simulink model "MTDC_MODEL"  (R2021a)
settings: Solver=ode1  StartTime=0.0  StopTime=3  FixedStep=2e-5  MaxStep=1e-5  RelTol=1e-5  EnableMultiTasking=on
InitFcn:
  | tau_iac=ts_G_iac/4;                                         %Current loop speed
  | wAC=1/tau_iac;                                              %Frequency
  | L1AC=wAC/s;                                                 %Open loop IMC (L) transfer function to obtain a first order after closing the loop
  | Kp_AC=wAC*(Lg_1+La_1/2);                                    %Proportional constant of the controller
  | Ki_AC=wAC*(Rg_1+Ra_1/2);                                    %Integral constant of the controller
  | C_IMC_AC=(Kp_AC*s+Ki_AC)/s;                                 %IMC designed PI controller transfer function
  | TAC=minreal((C_IMC_AC)*G_iac/(1+(C_IMC_AC)*G_iac));         %Closed loop transfer function
  | 
  | tau_Pac=ts_G_P/4;
  | D = TAC*U_ll1;
  | [C_pi,info] = pidtune(D,'PI',1/tau_Pac);
  | Ki_P = C_pi.Ki;
  | 
  | tau_Qac=ts_G_Q/4;
  | [C_piq,info] = pidtune(D,'PI',1/tau_Qac);
  | Ki_Q = C_piq.Ki;
  | 
  | 
  | tau_isum=ts_G_isum/4;                                        %Current loop speed
  | wsum=1/tau_isum;                                             %Frequency
  | L1AC=wsum/s;                                                 %Open loop IMC (L) transfer function to obtain a first order after closing the loop
  | Kp_sum=wsum*(2*La_1);                                        %Proportional constant of the controller
  | Ki_sum=wsum*(2*Ra_1);                                        %Integral constant of the controller
  | C_IMC_sum=(Kp_sum*s+Ki_sum)/s;                               %IMC designed PI controller transfer function
  | 
  | Kp_sum_PR = wc*(2*La_1);
  | Ki_sum_PR = wc*(2*Ra_1);
  | PR = (Kp_sum_PR*s^2 + 2*wc*(Kp_sum_PR+Ki_sum_PR)*s +Kp_sum_PR*w0^2)/(s^2+2*wc*s+w0^2);
  | 
  | 
  | %Energy reference for a converter arm (sum of all the submodule energies)
  | ArmEnergyRef=1/2*Carm*ArmVoltageRef^2;                      %Energy reference for a converter leg
  | LegEnergy=ArmEnergyRef*2;                                   %References for the controllers (DC side)
  | TotalEnergyRef=ArmEnergyRef*6;                              %Reference of the total energy of the converter
  | EnergyDiffabRef=0;                                          %Reference for the energy difference between legs a and b
  | EnergyDiffacRef=0;                                          %Reference for the energy difference between legs b and c
  | 
  | %References for the controllers (AC side)
  | EnergyDiffUpLowRefa=0;                                      %Reference for the energy difference upper and lower arms of phase a
  | EnergyDiffUpLowRefb=0;                                      %Reference for the energy difference upper and lower arms of phase b
  | EnergyDiffUpLowRefc=0;                                      %Reference for the energy difference upper and lower arms of phase c
  |                                                             %Controller design
  | Kpenergy=50;                                                %Proportional gain
  | Kienergy=20;                                                %Integral gain
  | 
  | Kpenergyt=50;                                               %Proportional gain
  | Kienergyt=20;                                               %Integral gain
  | 
  | Q=3;
  | wn=50*2*pi;                                                 %Frequency to eliminate 50 Hz
  | N_50 = tf([1 0 wn^2],[1 2*wn/Q wn^2]);                       %Notch filter 1 design
  | wn=100*2*pi;                                                %Frequency to eliminate 100 Hz
  | N_100 = tf([1 0 wn^2],[1 2*wn/Q wn^2]);                      %Notch filter 2 design
  | Notch=N_50*N_100;                                            %Combination of both notch filters
  | 
  | Ibasedc1= 1000e6/640e3;                 %Nominal current peak DC
  | IsaturationinnerDC1=1.1*Ibasedc1/3;  %Saturation of the DC inner current
  | IsaturationinnerAC1=0.45*Ibasedc1/3; %0.45  %Saturation of the inner current (why edu used 10% - FYI I changed it to 45%)
  | 
  | 
  | ... (+30 lines)
values from neighbouring files (symbols this model uses):
  ArmVoltageRef = 640e3    (= 640000)    [MMC_PARAMETERS.m]
  Cap = 9.5e-3    (= 0.0095)    [MMC_PARAMETERS.m]
  Carm = Cap/N    (= 2.375e-05)    [MMC_PARAMETERS.m]
  f_grid = 50    [MMC_PARAMETERS.m]
  La_1 = 0.15*Zbase_1/2/pi/50    (= 0.0488923985178)    [MMC_PARAMETERS.m]
  Lg_1 = 0.18*Zbase_1/2/pi/50    (= 0.0586708782214)    [MMC_PARAMETERS.m]
  N = 400    [MMC_PARAMETERS.m]
  Ra_1 = 0.01*Zbase_1    (= 1.024)    [MMC_PARAMETERS.m]
  Rg_1 = 0.005*Zbase_1    (= 0.512)    [MMC_PARAMETERS.m]
  S_1 = 1000e6    (= 1000000000)    [MMC_PARAMETERS.m]
  U_ll1 = 320e3    (= 320000)    [MMC_PARAMETERS.m]
  Vdc = 640e3    (= 640000)    [MMC_PARAMETERS.m]
  Vpeak_d1 = U_pnpeak1    [MMC_PARAMETERS.m]
  w0 = 2*pi*50    (= 314.159265359)    [MMC_PARAMETERS.m]
undefined symbols (not defined in the file or in its folder): Kp_Pac, lenght
libraries: spsSeriesRLCBranchLib x80, spsCurrentMeasurementLib x64, spsControlledVoltageSourceLib x36, pid_lib x32, spsVoltageMeasurementLib x32, spsControlledCurrentSourceLib x24, spsParallelRLCBranchLib x20, spsGroundLib x10, powerlib_extras x4, spsDCVoltageSourceLib x4, spspowerguiLib x1
(part 8 of 9)

== system MTDC_MODEL/GRID2+MMC2/Current loop1/Twisting ==
  iq : Inport
  Ref_iq : Inport  Port=2
  Ref_id : Inport  Port=3
  id : Inport  Port=4
  Add : Sum  Inputs=---
  Derivative2 : Derivative
  Gain1 : Gain  Gain=7500
  Gain2 : Gain  Gain=(Rg_1+Ra_1/2)
  Gain4 : Gain  Gain=1000
  Gain5 : Gain  Gain=(Lg_1+La_1/2)
  Gain6 : Gain  Gain=(Lg_1+La_1/2)*2*pi*50
  Scope : Scope  NumInputPorts=2
  Scope1 : Scope  NumInputPorts=2
  Sign : Signum  ZeroCross=off
  Sign1 : Signum  ZeroCross=off
  Sum2 : Sum  Inputs=|++
  Sum5 : Sum  Inputs=|+-
  Out1 : Outport
  Sq : Outport  Port=2
  wires:
  Gain5/1 -> Scope/2, Add/3
  Sign/1 -> Gain4/1
  Gain4/1 -> Sum2/1
  Sum2/1 -> Gain5/1
  Ref_iq/1 -> Gain2/1, Sum5/1
  Gain2/1 -> Add/2
  Gain6/1 -> Add/1
  Add/1 -> Out1/1, Scope/1
  iq/1 -> Sum5/2
  Sum5/1 -> Derivative2/1, Scope1/2, Sq/1, Sign/1  "Sq"
  Ref_id/1 -> Gain6/1
  Sign1/1 -> Gain1/1
  Derivative2/1 -> Sign1/1, Scope1/1
  Gain1/1 -> Sum2/2

== system MTDC_MODEL/GRID2+MMC2/DC References/Sat3 ==
  In1 : Inport
  Demux4 : Demux  Outputs=3
  Mux5 : Mux  Inputs=3
  Saturation1 : Saturate  UpperLimit=IsaturationinnerDC1  LowerLimit=-IsaturationinnerDC1
  Saturation4 : Saturate  UpperLimit=IsaturationinnerDC1  LowerLimit=-IsaturationinnerDC1
  Saturation5 : Saturate  UpperLimit=IsaturationinnerDC1  LowerLimit=-IsaturationinnerDC1
  Out1 : Outport  VectorParamsAs1DForOutWhenUnconnected=off
  wires:
  Saturation5/1 -> Mux5/3
  Saturation4/1 -> Mux5/2
  Saturation1/1 -> Mux5/1
  Demux4/3 -> Saturation5/1
  Demux4/2 -> Saturation4/1
  Demux4/1 -> Saturation1/1
  Mux5/1 -> Out1/1
  In1/1 -> Demux4/1

== system MTDC_MODEL/GRID2+MMC2/Energy Calculation1/AC Power Reference ==
  Ediff_arm_a : Inport
  Ediff_arm_b : Inport  Port=2
  Ediff_arm_c : Inport  Port=3
  Constant1 : Constant  Value=EnergyDiffUpLowRefb
  Constant2 : Constant  Value=EnergyDiffUpLowRefc
  Constant21 : Constant  Value=EnergyDiffUpLowRefa
  PI1 : TransferFcn  Numerator=[Notch.num{1}]  Denominator=[Notch.den{1}]
  PI2 : TransferFcn  Numerator=[Notch.num{1}]  Denominator=[Notch.den{1}]
  PI3 : Subsystem
  PI4 : Subsystem
  PI5 : Subsystem
  PI6 : TransferFcn  Numerator=[Notch.num{1}]  Denominator=[Notch.den{1}]
  Product : Product
  Step : Step  Time=2.1  Before=1  SampleTime=0
  Sum20 : Sum  Inputs=|+-
  Sum21 : Sum  Inputs=|+-
  Sum25 : Sum  Inputs=|+-
  Pdiff_arm_a_Ref : Outport  VectorParamsAs1DForOutWhenUnconnected=off
  Pdiff_arm_b_Ref : Outport  Port=2  VectorParamsAs1DForOutWhenUnconnected=off
  Pdiff_arm_c_Ref : Outport  Port=3  VectorParamsAs1DForOutWhenUnconnected=off
  wires:
  Constant21/1 -> Sum20/1
  Sum25/1 -> PI5/1(e)
  Constant1/1 -> Sum21/1
  Constant2/1 -> Sum25/1
  Sum21/1 -> PI4/1(e)
  Ediff_arm_c/1 -> Sum25/2
  Ediff_arm_a/1 -> Sum20/2
  PI6/1 -> Pdiff_arm_c_Ref/1
  PI5/1(u) -> PI6/1
  PI1/1 -> Pdiff_arm_a_Ref/1
  Sum20/1 -> Product/1
  Ediff_arm_b/1 -> Sum21/2
  PI2/1 -> Pdiff_arm_b_Ref/1
  PI3/1(u) -> PI1/1
  PI4/1(u) -> PI2/1
  Product/1 -> PI3/1(e)
  Step/1 -> Product/2

== system MTDC_MODEL/GRID2+MMC2/Energy Calculation1/DC Energy PIs ==
  EnergyTotal : Inport
  Energydiffab : Inport  Port=2
  Energydiffac : Inport  Port=3
  ACpowerFFd : Inport  Port=4
  DiffabABpowerFFd : Inport  Port=5
  DiffacACpowerFFd : Inport  Port=6
  Constant20 : Constant  Value=TotalEnergyRef
  Constant23 : Constant  Value=EnergyDiffabRef
  Constant29 : Constant  Value=EnergyDiffacRef
  Gain1 : Gain
  Gain43 : Gain
  Gain6 : Gain
  PI1 : TransferFcn  Numerator=[Notch.num{1}]  Denominator=[Notch.den{1}]
  PI10 : TransferFcn  Numerator=[Notch.num{1}]  Denominator=[Notch.den{1}]
  PI2 : TransferFcn  Numerator=[Notch.num{1}]  Denominator=[Notch.den{1}]
  PI3 : TransferFcn  Numerator=[Kpenergyt Kienergyt]  Denominator=[1 0 ]
  PI4 : TransferFcn  Numerator=[Kpenergyt Kienergyt]  Denominator=[1 0 ]
  PI5 : TransferFcn  Numerator=[Kpenergyt Kienergyt]  Denominator=[1 0 ]
  Sum10 : Sum  Inputs=|++
  Sum17 : Sum  Inputs=|++
  Sum20 : Sum  Inputs=|+-
  Sum21 : Sum  Inputs=|+-
  Sum25 : Sum  Inputs=|+-
  Sum27 : Sum  Inputs=|++
  TotalPowerRef : Outport  VectorParamsAs1DForOutWhenUnconnected=off
  DiffabPowerRef : Outport  Port=2  VectorParamsAs1DForOutWhenUnconnected=off
  DiffacPowerRef : Outport  Port=3  VectorParamsAs1DForOutWhenUnconnected=off
  wires:
  Constant20/1 -> Sum20/1
  Sum20/1 -> PI3/1
  Sum25/1 -> PI5/1
  Constant23/1 -> Sum21/1
  Constant29/1 -> Sum25/1
  Sum21/1 -> PI4/1
  PI5/1 -> Gain6/1
  Energydiffab/1 -> Sum21/2
  Energydiffac/1 -> Sum25/2
  EnergyTotal/1 -> Sum20/2
  PI3/1 -> Gain1/1
  PI4/1 -> Gain43/1
  PI2/1 -> DiffabPowerRef/1
  PI10/1 -> DiffacPowerRef/1
  Gain43/1 -> Sum10/1
  Sum17/1 -> PI10/1
  Gain6/1 -> Sum17/1
  Sum10/1 -> PI2/1
  ACpowerFFd/1 -> Sum27/2
  Gain1/1 -> Sum27/1
  PI1/1 -> TotalPowerRef/1
  Sum27/1 -> PI1/1
  DiffacACpowerFFd/1 -> Sum17/2
  DiffabABpowerFFd/1 -> Sum10/2

== system MTDC_MODEL/GRID2+MMC2/Feedforward calculation/First order filter1 ==
  In1 : Inport
  Demux11 : Demux  Outputs=3
  Mux23 : Mux  Inputs=3
  R1 : TransferFcn  Numerator=1  Denominator=[tau_isum 1]
  R2 : TransferFcn  Numerator=1  Denominator=[tau_isum 1]
  R3 : TransferFcn  Numerator=1  Denominator=[tau_isum 1]
  Out1 : Outport  VectorParamsAs1DForOutWhenUnconnected=off
  wires:
  Demux11/2 -> R2/1
  R2/1 -> Mux23/2  "Pub"
  Demux11/1 -> R1/1
  Demux11/3 -> R3/1
  Mux23/1 -> Out1/1
  In1/1 -> Demux11/1
  R3/1 -> Mux23/3  "Puc"
  R1/1 -> Mux23/1  "Pua"

== system MTDC_MODEL/GRID2+MMC2/Isum_AC_Ref_Cal/DIFFERENT_REF_CALC_METHODS  ==
  v_g_pos : Inport
  Constant{1..6} (6 alike) : Constant  Value=0
  Gain1 : Gain  Gain=1/sqrt(2)
  Gain13 : Gain  Gain=1/U_ll1
  Matrix Concatenate4 : Concatenate  NumInputs=3  Mode=Multidimensional array  ConcatenateDimension=2
  Memory : Memory  InitialCondition=Vpeak_d1
  Mux11 : Mux  Inputs=3
  Mux12 : Mux  Inputs=3
  Mux5 : Mux  Inputs=3
  inv mat2 : MATLAB Function  TreatAsAtomicUnit=on
  Initial Approach : Outport  VectorParamsAs1DForOutWhenUnconnected=off
  wires:
  Mux5/1 -> Matrix Concatenate4/3
  Mux11/1 -> Matrix Concatenate4/1
  Constant5/1 -> Mux11/2
  Matrix Concatenate4/1 -> inv mat2/1(u)  "Isum_neg; -Isum_neg;  Isum_pos"
  Constant4/1 -> Mux12/1
  [v_g_pos_rms_pu] -> Mux11/1
  [v_g_pos_rms_pu] -> Mux12/2
  Constant3/1 -> Mux5/2
  [v_g_pos_rms_pu] -> Mux5/3
  inv mat2/1(y) -> Initial Approach/1
  Mux12/1 -> Matrix Concatenate4/2
  Gain1/1 -> [v_g_pos_rms_pu]
  v_g_pos/1 -> Memory/1
  Gain13/1 -> Gain1/1
  Constant1/1 -> Mux11/3
  Constant2/1 -> Mux12/3
  Constant6/1 -> Mux5/1
  Memory/1 -> Gain13/1

== system MTDC_MODEL/GRID2+MMC2/Isum_AC_Ref_Cal/Rotation4 ==
  angle : Inport
  Gain1 : Gain
  Gain2 : Gain  Gain=-1
  Gain9 : Gain  Gain=-1
  Matrix Concatenate1 : Concatenate  Mode=Multidimensional array  ConcatenateDimension=2
  Matrix Concatenate2 : Concatenate  Mode=Multidimensional array  ConcatenateDimension=2
  Mux{1..2,8..9} (4 alike) : Mux  Inputs=2
  Trigonometric Function{1,3..4,6} (4 alike) : Trigonometry  Operator=cos
  Trigonometric Function{2,5,7..8} (4 alike) : Trigonometry
  iR : Outport  VectorParamsAs1DForOutWhenUnconnected=off
  R : Outport  Port=2  VectorParamsAs1DForOutWhenUnconnected=off
  wires:
  Gain2/1 -> Mux2/1
  Matrix Concatenate2/1 -> R/1
  Gain1/1 -> Mux1/2
  Mux2/1 -> Matrix Concatenate2/2
  Mux1/1 -> Matrix Concatenate2/1
  Trigonometric Function8/1 -> Gain2/1
  Trigonometric Function2/1 -> Gain1/1
  Trigonometric Function3/1 -> Mux2/2
  Trigonometric Function1/1 -> Mux1/1
  Matrix Concatenate1/1 -> iR/1
  Gain9/1 -> Mux8/2
  angle/1 -> Trigonometric Function1/1, Trigonometric Function2/1, Trigonometric Function8/1, Trigonometric Function3/1, Trigonometric Function4/1, Trigonometric Function5/1, Trigonometric Function7/1, Trigonometric Function6/1
  Mux9/1 -> Matrix Concatenate1/2
  Mux8/1 -> Matrix Concatenate1/1
  Trigonometric Function7/1 -> Mux9/1
  Trigonometric Function5/1 -> Gain9/1
  Trigonometric Function6/1 -> Mux9/2
  Trigonometric Function4/1 -> Mux8/1

== system MTDC_MODEL/GRID2+MMC2/vsum Calculation/PR Controller1 ==
  e : Inport
  PID Controller2 : pid_lib/PID Controller  Controller=PI  Form=Parallel  TimeDomain=Continuous-time  UseExternalTs=off  SampleTime=1  IntegratorMethod=Forward Euler  FilterMethod=Forward Euler  ControllerParametersSource=internal  P=Kp_sum  I=Ki_sum  D=0  UseFilter=on  N=100  TunerSelectOption=Transfer Function Based (PID Tuner App)  InitialConditionSource=internal  InitialConditionForIntegrator=0  InitialConditionForFilter=0  DifferentiatorICPrevScaledInput=0  ExternalReset=none  TrackingMode=off  Kt=1  LimitOutput=off  SatLimitsSource=internal  UpperSaturationLimit=inf  LowerSaturationLimit=-inf  LinearizeAsGain=on  AntiWindupMode=none  Kb=1  POutMin=[]  POutMax=[]  IOutMin=[]  IOutMax=[]  DOutMin=[]  DOutMax=[]  NOutMin=[]  NOutMax=[]  SumOutMin=[]  SumOutMax=[]  SaturationOutMin=[]  SaturationOutMax=[]  PParamMin=[]  PParamMax=[]  IParamMin=[]  IParamMax=[]  DParamMin=[]  DParamMax=[]  NParamMin=[]  NParamMax=[]  KbParamMin=[]  KbParamMax=[]  KtParamMin=[]  KtParamMax=[]  KbOutMin=[]  KbOutMax=[]  KtOutMin=[]  KtOutMax=[]  IntegratorOutMin=[]  IntegratorOutMax=[]  FilterOutMin=[]  FilterOutMax=[]  SumI1OutMin=[]  SumI1OutMax=[]  SumI2OutMin=[]  SumI2OutMax=[]  SumI3OutMin=[]  SumI3OutMax=[]  SumI4OutMin=[]  SumI4OutMax=[]  SumDOutMin=[]  SumDOutMax=[]  DifferentiatorOutMin=[]  DifferentiatorOutMax=[]  FilterDiffOutCoefMin=[]  FilterDiffOutCoefMax=[]  ReciprocalOutMin=[]  ReciprocalOutMax=[]  SumDenOutMin=[]  SumDenOutMax=[]  SumNumOutMin=[]  SumNumOutMax=[]  DivideOutMin=[]  DivideOutMax=[]  UdiffTsProdOutMin=[]  UdiffTsProdOutMax=[]  NTsProdOutMin=[]  NTsProdOutMax=[]  UintegralTsProdOutMin=[]  UintegralTsProdOutMax=[]  UngainTsProdOutMin=[]  UngainTsProdOutMax=[]  IntegratorContinuousStateAttributes=''  IntegratorStateMustResolveToSignalObject=off  IntegratorRTWStateStorageClass=Auto  FilterContinuousStateAttributes=''  FilterStateMustResolveToSignalObject=off  FilterRTWStateStorageClass=Auto  ParallelPVariant=InternalParameters  IdealPVariant=Disabled  IVariant=InternalParameters  DVariant=Disabled  IntegratorVariant=Continuous  SatVariant=Disabled  AWVariant=Passthrough  PCopyVariant=Disabled  TRVariant=Disabled  FdbkBlocksVariant=Forward  IdealPFdbkVariant=Disabled  SatFdbkVariant=Disabled  DerivativeFilterVariant=Disabled  NVariant=Disabled  NCopyVariant=Disabled_SignalSpec  FilterICVariant=Disabled  IntegratorICVariant=InternalICs  ExternalResetVariant=Disabled  TRSumVariant=Passthrough  SumFdbkVariant=Disabled  SumVariant=Sum_PI  TsampFilterVariant=InternalTs  TsampNgainVariant=Passthrough  TsampIntegralVariant=Passthrough  ExternalSaturationOutDataTypeStr=Inherit: Same as second input
  Sum1 : Sum  Inputs=++|
  Transfer Fcn : TransferFcn  Numerator=PR.num{1}  Denominator=PR.den{1}
  v : Outport
  wires:
  e/1 -> Transfer Fcn/1, PID Controller2/1
  Transfer Fcn/1 -> Sum1/2
  Sum1/1 -> v/1
  PID Controller2/1 -> Sum1/1

== system MTDC_MODEL/GRID2+MMC2/vsum Calculation/PR Controller2 ==
  e : Inport
  PID Controller2 : pid_lib/PID Controller  Controller=PI  Form=Parallel  TimeDomain=Continuous-time  UseExternalTs=off  SampleTime=1  IntegratorMethod=Forward Euler  FilterMethod=Forward Euler  ControllerParametersSource=internal  P=Kp_sum  I=Ki_sum  D=0  UseFilter=on  N=100  TunerSelectOption=Transfer Function Based (PID Tuner App)  InitialConditionSource=internal  InitialConditionForIntegrator=0  InitialConditionForFilter=0  DifferentiatorICPrevScaledInput=0  ExternalReset=none  TrackingMode=off  Kt=1  LimitOutput=off  SatLimitsSource=internal  UpperSaturationLimit=inf  LowerSaturationLimit=-inf  LinearizeAsGain=on  AntiWindupMode=none  Kb=1  POutMin=[]  POutMax=[]  IOutMin=[]  IOutMax=[]  DOutMin=[]  DOutMax=[]  NOutMin=[]  NOutMax=[]  SumOutMin=[]  SumOutMax=[]  SaturationOutMin=[]  SaturationOutMax=[]  PParamMin=[]  PParamMax=[]  IParamMin=[]  IParamMax=[]  DParamMin=[]  DParamMax=[]  NParamMin=[]  NParamMax=[]  KbParamMin=[]  KbParamMax=[]  KtParamMin=[]  KtParamMax=[]  KbOutMin=[]  KbOutMax=[]  KtOutMin=[]  KtOutMax=[]  IntegratorOutMin=[]  IntegratorOutMax=[]  FilterOutMin=[]  FilterOutMax=[]  SumI1OutMin=[]  SumI1OutMax=[]  SumI2OutMin=[]  SumI2OutMax=[]  SumI3OutMin=[]  SumI3OutMax=[]  SumI4OutMin=[]  SumI4OutMax=[]  SumDOutMin=[]  SumDOutMax=[]  DifferentiatorOutMin=[]  DifferentiatorOutMax=[]  FilterDiffOutCoefMin=[]  FilterDiffOutCoefMax=[]  ReciprocalOutMin=[]  ReciprocalOutMax=[]  SumDenOutMin=[]  SumDenOutMax=[]  SumNumOutMin=[]  SumNumOutMax=[]  DivideOutMin=[]  DivideOutMax=[]  UdiffTsProdOutMin=[]  UdiffTsProdOutMax=[]  NTsProdOutMin=[]  NTsProdOutMax=[]  UintegralTsProdOutMin=[]  UintegralTsProdOutMax=[]  UngainTsProdOutMin=[]  UngainTsProdOutMax=[]  IntegratorContinuousStateAttributes=''  IntegratorStateMustResolveToSignalObject=off  IntegratorRTWStateStorageClass=Auto  FilterContinuousStateAttributes=''  FilterStateMustResolveToSignalObject=off  FilterRTWStateStorageClass=Auto  ParallelPVariant=InternalParameters  IdealPVariant=Disabled  IVariant=InternalParameters  DVariant=Disabled  IntegratorVariant=Continuous  SatVariant=Disabled  AWVariant=Passthrough  PCopyVariant=Disabled  TRVariant=Disabled  FdbkBlocksVariant=Forward  IdealPFdbkVariant=Disabled  SatFdbkVariant=Disabled  DerivativeFilterVariant=Disabled  NVariant=Disabled  NCopyVariant=Disabled_SignalSpec  FilterICVariant=Disabled  IntegratorICVariant=InternalICs  ExternalResetVariant=Disabled  TRSumVariant=Passthrough  SumFdbkVariant=Disabled  SumVariant=Sum_PI  TsampFilterVariant=InternalTs  TsampNgainVariant=Passthrough  TsampIntegralVariant=Passthrough  ExternalSaturationOutDataTypeStr=Inherit: Same as second input
  Sum1 : Sum  Inputs=++|
  Transfer Fcn : TransferFcn  Numerator=PR.num{1}  Denominator=PR.den{1}
  v : Outport
  wires:
  PID Controller2/1 -> Sum1/1
  Sum1/1 -> v/1
  Transfer Fcn/1 -> Sum1/2
  e/1 -> PID Controller2/1, Transfer Fcn/1

== system MTDC_MODEL/GRID2+MMC2/vsum Calculation/PR Controller3 ==
  e : Inport
  PID Controller2 : pid_lib/PID Controller  Controller=PI  Form=Parallel  TimeDomain=Continuous-time  UseExternalTs=off  SampleTime=1  IntegratorMethod=Forward Euler  FilterMethod=Forward Euler  ControllerParametersSource=internal  P=Kp_sum  I=Ki_sum  D=0  UseFilter=on  N=100  TunerSelectOption=Transfer Function Based (PID Tuner App)  InitialConditionSource=internal  InitialConditionForIntegrator=0  InitialConditionForFilter=0  DifferentiatorICPrevScaledInput=0  ExternalReset=none  TrackingMode=off  Kt=1  LimitOutput=off  SatLimitsSource=internal  UpperSaturationLimit=inf  LowerSaturationLimit=-inf  LinearizeAsGain=on  AntiWindupMode=none  Kb=1  POutMin=[]  POutMax=[]  IOutMin=[]  IOutMax=[]  DOutMin=[]  DOutMax=[]  NOutMin=[]  NOutMax=[]  SumOutMin=[]  SumOutMax=[]  SaturationOutMin=[]  SaturationOutMax=[]  PParamMin=[]  PParamMax=[]  IParamMin=[]  IParamMax=[]  DParamMin=[]  DParamMax=[]  NParamMin=[]  NParamMax=[]  KbParamMin=[]  KbParamMax=[]  KtParamMin=[]  KtParamMax=[]  KbOutMin=[]  KbOutMax=[]  KtOutMin=[]  KtOutMax=[]  IntegratorOutMin=[]  IntegratorOutMax=[]  FilterOutMin=[]  FilterOutMax=[]  SumI1OutMin=[]  SumI1OutMax=[]  SumI2OutMin=[]  SumI2OutMax=[]  SumI3OutMin=[]  SumI3OutMax=[]  SumI4OutMin=[]  SumI4OutMax=[]  SumDOutMin=[]  SumDOutMax=[]  DifferentiatorOutMin=[]  DifferentiatorOutMax=[]  FilterDiffOutCoefMin=[]  FilterDiffOutCoefMax=[]  ReciprocalOutMin=[]  ReciprocalOutMax=[]  SumDenOutMin=[]  SumDenOutMax=[]  SumNumOutMin=[]  SumNumOutMax=[]  DivideOutMin=[]  DivideOutMax=[]  UdiffTsProdOutMin=[]  UdiffTsProdOutMax=[]  NTsProdOutMin=[]  NTsProdOutMax=[]  UintegralTsProdOutMin=[]  UintegralTsProdOutMax=[]  UngainTsProdOutMin=[]  UngainTsProdOutMax=[]  IntegratorContinuousStateAttributes=''  IntegratorStateMustResolveToSignalObject=off  IntegratorRTWStateStorageClass=Auto  FilterContinuousStateAttributes=''  FilterStateMustResolveToSignalObject=off  FilterRTWStateStorageClass=Auto  ParallelPVariant=InternalParameters  IdealPVariant=Disabled  IVariant=InternalParameters  DVariant=Disabled  IntegratorVariant=Continuous  SatVariant=Disabled  AWVariant=Passthrough  PCopyVariant=Disabled  TRVariant=Disabled  FdbkBlocksVariant=Forward  IdealPFdbkVariant=Disabled  SatFdbkVariant=Disabled  DerivativeFilterVariant=Disabled  NVariant=Disabled  NCopyVariant=Disabled_SignalSpec  FilterICVariant=Disabled  IntegratorICVariant=InternalICs  ExternalResetVariant=Disabled  TRSumVariant=Passthrough  SumFdbkVariant=Disabled  SumVariant=Sum_PI  TsampFilterVariant=InternalTs  TsampNgainVariant=Passthrough  TsampIntegralVariant=Passthrough  ExternalSaturationOutDataTypeStr=Inherit: Same as second input
  Sum1 : Sum  Inputs=++|
  Transfer Fcn : TransferFcn  Numerator=PR.num{1}  Denominator=PR.den{1}
  v : Outport
  wires:
  e/1 -> Transfer Fcn/1, PID Controller2/1
  Transfer Fcn/1 -> Sum1/2
  Sum1/1 -> v/1
  PID Controller2/1 -> Sum1/1

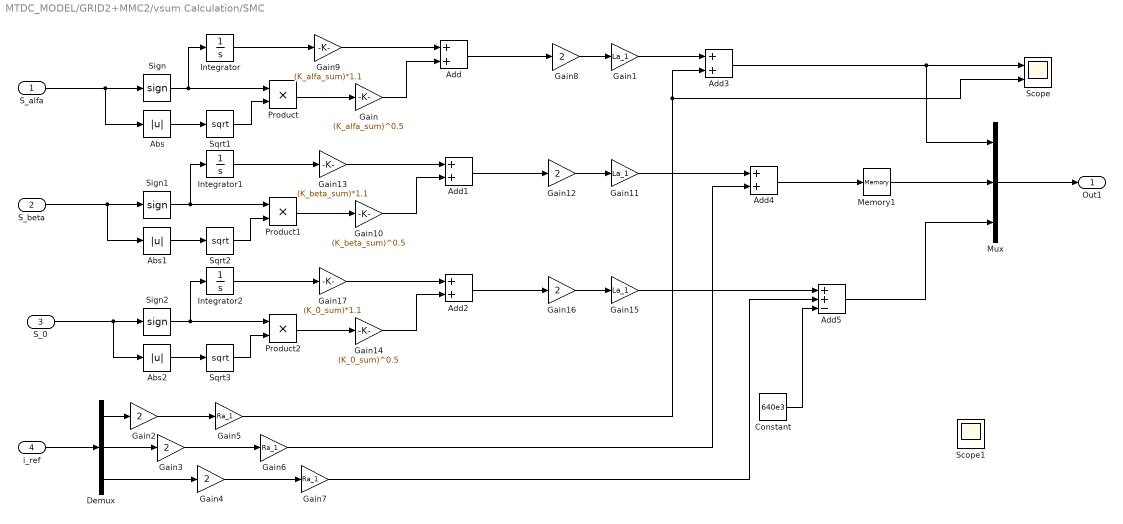
== system MTDC_MODEL/GRID2+MMC2/vsum Calculation/SMC ==
  S_alfa : Inport
  S_beta : Inport  Port=2
  S_0 : Inport  Port=3
  i_ref : Inport  Port=4
  Abs : Abs
  Abs1 : Abs
  Abs2 : Abs
  Add{,1..4} (5 alike) : Sum
  Add5 : Sum  Inputs=++-
  Constant : Constant  Value=640e3
  Demux : Demux  Outputs=3
  Gain : Gain  Gain=(K_alfa_sum)^0.5
  Gain1 : Gain  Gain=La_1
  Gain10 : Gain  Gain=(K_beta_sum)^0.5
  Gain11 : Gain  Gain=La_1
  Gain{2..4,8,12,16} (6 alike) : Gain  Gain=2
  Gain13 : Gain  Gain=(K_beta_sum)*1.1
  Gain14 : Gain  Gain=(K_0_sum)^0.5
  Gain15 : Gain  Gain=La_1
  Gain17 : Gain  Gain=(K_0_sum)*1.1
  Gain5 : Gain  Gain=Ra_1
  Gain6 : Gain  Gain=Ra_1
  Gain7 : Gain  Gain=Ra_1
  Gain9 : Gain  Gain=(K_alfa_sum)*1.1
  Integrator : Integrator
  Integrator1 : Integrator
  Integrator2 : Integrator
  Memory1 : Memory
  Mux : Mux  Inputs=3
  Product : Product
  Product1 : Product
  Product2 : Product
  Scope : Scope  NumInputPorts=2
  Scope1 : Scope
  Sign : Signum
  Sign1 : Signum
  Sign2 : Signum
  Sqrt1 : Sqrt  SaturateOnIntegerOverflow=on
  Sqrt2 : Sqrt  SaturateOnIntegerOverflow=on
  Sqrt3 : Sqrt  SaturateOnIntegerOverflow=on
  Out1 : Outport
  wires:
  i_ref/1 -> Demux/1
  Demux/1 -> Gain2/1
  Demux/2 -> Gain3/1
  Demux/3 -> Gain4/1
  Gain2/1 -> Gain5/1
  Gain3/1 -> Gain6/1
  Gain4/1 -> Gain7/1
  Gain8/1 -> Gain1/1
  S_alfa/1 -> Abs/1, Sign/1
  Sign/1 -> Integrator/1, Product/1
  Product/1 -> Gain/1
  Abs/1 -> Sqrt1/1
  Sqrt1/1 -> Product/2
  Integrator/1 -> Gain9/1
  Gain/1 -> Add/2
  Gain9/1 -> Add/1
  Add/1 -> Gain8/1
  Add1/1 -> Gain12/1
  Gain13/1 -> Add1/1
  Gain10/1 -> Add1/2
  Integrator1/1 -> Gain13/1
  Sqrt2/1 -> Product1/2
  Abs1/1 -> Sqrt2/1
  Product1/1 -> Gain10/1
  Sign1/1 -> Integrator1/1, Product1/1
  S_beta/1 -> Sign1/1, Abs1/1
  Gain12/1 -> Gain11/1
  Gain16/1 -> Gain15/1
  Sign2/1 -> Integrator2/1, Product2/1
  Product2/1 -> Gain14/1
  Abs2/1 -> Sqrt3/1
  Sqrt3/1 -> Product2/2
  Integrator2/1 -> Gain17/1
  Gain14/1 -> Add2/2
  Gain17/1 -> Add2/1
  Add2/1 -> Gain16/1
  Gain6/1 -> Add4/2
  Gain1/1 -> Add3/1
  Gain11/1 -> Add4/1
  Mux/1 -> Out1/1
  Add4/1 -> Memory1/1
  Add5/1 -> Mux/3
  Memory1/1 -> Mux/2
  Gain15/1 -> Add5/1
  Gain7/1 -> Add5/2
  Gain5/1 -> Scope/2, Add3/2
  Add3/1 -> Scope/1, Mux/1
  S_0/1 -> Abs2/1, Sign2/1
  Constant/1 -> Add5/3

== system MTDC_MODEL/GRID3+MMC3/Current loop1/PLCS ==
  iq : Inport
  Ref_iq : Inport  Port=2
  Ref_id : Inport  Port=3
  id : Inport  Port=4
  Abs2 : Abs
  Add : Sum  Inputs=---
  Add1 : Sum
  Constant : Constant  Value=-1/5
  Derivative : Derivative
  Gain1 : Gain  Gain=20000
  Gain14 : Gain  Gain=3900
  Gain2 : Gain  Gain=(Rg_1+Ra_1/2)
  Gain3 : Gain  Gain=(Lg_1+La_1/2)
  Gain6 : Gain  Gain=(Lg_1+La_1/2)*2*pi*50
  Power : Math  Operator=pow  SaturateOnIntegerOverflow=on
  Power1 : Math  Operator=pow  SaturateOnIntegerOverflow=on
  Product : Product
  Scope : Scope  NumInputPorts=2
  Sign1 : Signum
  Sign2 : Signum
  Sqrt3 : Sqrt  SaturateOnIntegerOverflow=on
  Sum5 : Sum  Inputs=|+-
  Out1 : Outport
  Sq : Outport  Port=2
  wires:
  Ref_id/1 -> Gain6/1
  Sum5/1 -> Sign1/1, Scope/2, Sq/1, Derivative/1, Abs2/1  "Sq"
  iq/1 -> Sum5/2
  Add/1 -> Out1/1
  Gain6/1 -> Add/1
  Gain2/1 -> Add/2
  Ref_iq/1 -> Gain2/1, Sum5/1
  Gain3/1 -> Scope/1, Add/3
  Abs2/1 -> Sqrt3/1
  Sign1/1 -> Product/1
  Sqrt3/1 -> Product/2
  Product/1 -> Gain14/1
  Gain14/1 -> Add1/1
  Derivative/1 -> Add1/2
  Add1/1 -> Sign2/1
  Gain1/1 -> Gain3/1
  Sign2/1 -> Gain1/1

== system MTDC_MODEL/GRID3+MMC3/Current loop1/SMC ==
  iq : Inport
  Ref_iq : Inport  Port=2
  Ref_id : Inport  Port=3
  id : Inport  Port=4
  Add : Sum  Inputs=---
  Gain2 : Gain  Gain=(Rg_1+Ra_1/2)
  Gain3 : Gain  Gain=Kq
  Gain4 : Gain  Gain=Qq
  Gain5 : Gain  Gain=(Lg_1+La_1/2)
  Gain6 : Gain  Gain=(Lg_1+La_1/2)*2*pi*50
  Sign : Signum  ZeroCross=off
  Sum2 : Sum  Inputs=|++
  Sum5 : Sum  Inputs=|+-
  Out1 : Outport
  Sq : Outport  Port=2
  wires:
  Sign/1 -> Gain4/1
  Gain3/1 -> Sum2/2
  Gain4/1 -> Sum2/1
  Sum2/1 -> Gain5/1
  Ref_iq/1 -> Gain2/1, Sum5/1
  Gain5/1 -> Add/3
  Gain2/1 -> Add/2
  Gain6/1 -> Add/1
  Add/1 -> Out1/1
  iq/1 -> Sum5/2
  Sum5/1 -> Sq/1, Gain3/1, Sign/1  "Sq"
  Ref_id/1 -> Gain6/1

== system MTDC_MODEL/GRID3+MMC3/Current loop1/SMC1 ==
  id : Inport
  Ref_id : Inport  Port=2
  Ref_iq : Inport  Port=3
  iq : Inport  Port=4
  Add : Sum  Inputs=+--
  Gain2 : Gain  Gain=(Rg_1+Ra_1/2)
  Gain3 : Gain  Gain=Kd
  Gain4 : Gain  Gain=Qd
  Gain5 : Gain  Gain=(Lg_1+La_1/2)
  Gain6 : Gain  Gain=(Lg_1+La_1/2)*2*pi*50
  Sign : Signum  ZeroCross=off
  Sum2 : Sum  Inputs=|++
  Sum5 : Sum  Inputs=|+-
  Out1 : Outport
  Sd : Outport  Port=2
  wires:
  Sum2/1 -> Gain5/1
  Gain4/1 -> Sum2/1
  Gain3/1 -> Sum2/2
  Sign/1 -> Gain4/1
  Ref_id/1 -> Gain2/1, Sum5/1
  Gain6/1 -> Add/1
  Gain2/1 -> Add/2
  Gain5/1 -> Add/3
  id/1 -> Sum5/2
  Sum5/1 -> Sd/1, Gain3/1, Sign/1  "Sd"
  Add/1 -> Out1/1
  Ref_iq/1 -> Gain6/1

== system MTDC_MODEL/GRID3+MMC3/Current loop1/ST-SMC ==
  iq : Inport
  Ref_iq : Inport  Port=2
  Ref_id : Inport  Port=3
  id : Inport  Port=4
  Abs2 : Abs
  Add : Sum  Inputs=---
  Add1 : Sum
  Gain14 : Gain  Gain=4000
  Gain17 : Gain  Gain=4000
  Gain2 : Gain  Gain=(Rg_1+Ra_1/2)
  Gain5 : Gain  Gain=(Lg_1+La_1/2)
  Gain6 : Gain  Gain=(Lg_1+La_1/2)*2*pi*50
  Integrator2 : Integrator
  Product2 : Product
  Scope : Scope  NumInputPorts=2
  Sign2 : Signum
  Sqrt3 : Sqrt  SaturateOnIntegerOverflow=on
  Sum5 : Sum  Inputs=|+-
  Out1 : Outport
  Sq : Outport  Port=2
  wires:
  Gain5/1 -> Scope/2, Add/3
  Ref_iq/1 -> Sum5/1, Gain2/1
  Gain2/1 -> Add/2
  Gain6/1 -> Add/1
  Add/1 -> Scope/1, Out1/1
  iq/1 -> Sum5/2
  Sum5/1 -> Sq/1, Abs2/1, Sign2/1  "Sq"
  Ref_id/1 -> Gain6/1
  Sign2/1 -> Integrator2/1, Product2/1
  Product2/1 -> Gain14/1
  Sqrt3/1 -> Product2/2
  Abs2/1 -> Sqrt3/1
  Integrator2/1 -> Gain17/1
  Add1/1 -> Gain5/1
  Gain17/1 -> Add1/1
  Gain14/1 -> Add1/2

== system MTDC_MODEL/GRID3+MMC3/Current loop1/Twisting ==
  iq : Inport
  Ref_iq : Inport  Port=2
  Ref_id : Inport  Port=3
  id : Inport  Port=4
  Add : Sum  Inputs=---
  Derivative2 : Derivative
  Gain1 : Gain  Gain=7500
  Gain2 : Gain  Gain=(Rg_1+Ra_1/2)
  Gain4 : Gain  Gain=1000
  Gain5 : Gain  Gain=(Lg_1+La_1/2)
  Gain6 : Gain  Gain=(Lg_1+La_1/2)*2*pi*50
  Scope : Scope  NumInputPorts=2
  Scope1 : Scope  NumInputPorts=2
  Sign : Signum  ZeroCross=off
  Sign1 : Signum  ZeroCross=off
  Sum2 : Sum  Inputs=|++
  Sum5 : Sum  Inputs=|+-
  To File1 : ToFile  Filename=sdot2.mat  MatrixName=ans_sdot2  SaveFormat=Timeseries
  To File6 : ToFile  Filename=s2.mat  MatrixName=ans_s2  SaveFormat=Timeseries
  Out1 : Outport
  Sq : Outport  Port=2
  wires:
  Gain5/1 -> Scope/2, Add/3
  Sign/1 -> Gain4/1
  Gain4/1 -> Sum2/1
  Sum2/1 -> Gain5/1
  Ref_iq/1 -> Gain2/1, Sum5/1
  Gain2/1 -> Add/2
  Gain6/1 -> Add/1
  Add/1 -> Out1/1, Scope/1
  iq/1 -> Sum5/2
  Sum5/1 -> Derivative2/1, To File6/1, Scope1/2, Sq/1, Sign/1  "Sq"
  Ref_id/1 -> Gain6/1
  Sign1/1 -> Gain1/1
  Derivative2/1 -> Sign1/1, To File1/1, Scope1/1
  Gain1/1 -> Sum2/2

== system MTDC_MODEL/GRID3+MMC3/DC References/Sat3 ==
  In1 : Inport
  Demux4 : Demux  Outputs=3
  Mux5 : Mux  Inputs=3
  Saturation1 : Saturate  UpperLimit=IsaturationinnerDC1  LowerLimit=-IsaturationinnerDC1
  Saturation4 : Saturate  UpperLimit=IsaturationinnerDC1  LowerLimit=-IsaturationinnerDC1
  Saturation5 : Saturate  UpperLimit=IsaturationinnerDC1  LowerLimit=-IsaturationinnerDC1
  Out1 : Outport  VectorParamsAs1DForOutWhenUnconnected=off
  wires:
  Saturation5/1 -> Mux5/3
  Saturation4/1 -> Mux5/2
  Saturation1/1 -> Mux5/1
  Demux4/3 -> Saturation5/1
  Demux4/2 -> Saturation4/1
  Demux4/1 -> Saturation1/1
  Mux5/1 -> Out1/1
  In1/1 -> Demux4/1

== system MTDC_MODEL/GRID3+MMC3/Energy Calculation1/AC Power Reference ==
  Ediff_arm_a : Inport
  Ediff_arm_b : Inport  Port=2
  Ediff_arm_c : Inport  Port=3
  Constant1 : Constant  Value=EnergyDiffUpLowRefb
  Constant2 : Constant  Value=EnergyDiffUpLowRefc
  Constant21 : Constant  Value=EnergyDiffUpLowRefa
  Mux : Mux  Inputs=3
  PI1 : TransferFcn  Numerator=[Notch.num{1}]  Denominator=[Notch.den{1}]
  PI2 : TransferFcn  Numerator=[Notch.num{1}]  Denominator=[Notch.den{1}]
  PI3 : Subsystem
  PI4 : Subsystem
  PI5 : Subsystem
  PI6 : TransferFcn  Numerator=[Notch.num{1}]  Denominator=[Notch.den{1}]
  Product : Product
  Scope : Scope
  Step : Step  Time=2.1  Before=1  SampleTime=0
  Sum20 : Sum  Inputs=|+-
  Sum21 : Sum  Inputs=|+-
  Sum25 : Sum  Inputs=|+-
  Pdiff_arm_a_Ref : Outport  VectorParamsAs1DForOutWhenUnconnected=off
  Pdiff_arm_b_Ref : Outport  Port=2  VectorParamsAs1DForOutWhenUnconnected=off
  Pdiff_arm_c_Ref : Outport  Port=3  VectorParamsAs1DForOutWhenUnconnected=off
  wires:
  Constant21/1 -> Sum20/1
  Sum25/1 -> PI5/1(e)
  Constant1/1 -> Sum21/1
  Constant2/1 -> Sum25/1
  Sum21/1 -> PI4/1(e)
  Ediff_arm_c/1 -> Mux/3, Sum25/2
  Ediff_arm_a/1 -> Mux/1, Sum20/2
  PI6/1 -> Pdiff_arm_c_Ref/1
  PI5/1(u) -> PI6/1
  PI1/1 -> Pdiff_arm_a_Ref/1
  Sum20/1 -> Product/1
  Ediff_arm_b/1 -> Mux/2, Sum21/2
  PI2/1 -> Pdiff_arm_b_Ref/1
  PI3/1(u) -> PI1/1
  PI4/1(u) -> PI2/1
  Product/1 -> PI3/1(e)
  Step/1 -> Product/2
  Mux/1 -> Scope/1

== system MTDC_MODEL/GRID3+MMC3/Energy Calculation1/DC Energy PIs ==
  EnergyTotal : Inport
  Energydiffab : Inport  Port=2
  Energydiffac : Inport  Port=3
  ACpowerFFd : Inport  Port=4
  DiffabABpowerFFd : Inport  Port=5
  DiffacACpowerFFd : Inport  Port=6
  Constant20 : Constant  Value=TotalEnergyRef
  Constant23 : Constant  Value=EnergyDiffabRef
  Constant29 : Constant  Value=EnergyDiffacRef
  Gain1 : Gain
  Gain43 : Gain
  Gain6 : Gain
  Mux : Mux  Inputs=2
  PI1 : TransferFcn  Numerator=[Notch.num{1}]  Denominator=[Notch.den{1}]
  PI10 : TransferFcn  Numerator=[Notch.num{1}]  Denominator=[Notch.den{1}]
  PI2 : TransferFcn  Numerator=[Notch.num{1}]  Denominator=[Notch.den{1}]
  PI3 : TransferFcn  Numerator=[Kpenergyt Kienergyt]  Denominator=[1 0 ]
  PI4 : TransferFcn  Numerator=[Kpenergyt Kienergyt]  Denominator=[1 0 ]
  PI5 : TransferFcn  Numerator=[Kpenergyt Kienergyt]  Denominator=[1 0 ]
  Scope : Scope
  Sum10 : Sum  Inputs=|++
  Sum17 : Sum  Inputs=|++
  Sum20 : Sum  Inputs=|+-
  Sum21 : Sum  Inputs=|+-
  Sum25 : Sum  Inputs=|+-
  Sum27 : Sum  Inputs=|++
  TotalPowerRef : Outport  VectorParamsAs1DForOutWhenUnconnected=off
  DiffabPowerRef : Outport  Port=2  VectorParamsAs1DForOutWhenUnconnected=off
  DiffacPowerRef : Outport  Port=3  VectorParamsAs1DForOutWhenUnconnected=off
  wires:
  Constant20/1 -> Sum20/1
  Sum20/1 -> PI3/1
  Sum25/1 -> PI5/1
  Constant23/1 -> Sum21/1
  Constant29/1 -> Sum25/1
  Sum21/1 -> PI4/1
  PI5/1 -> Gain6/1
  Energydiffab/1 -> Mux/1, Sum21/2
  Energydiffac/1 -> Mux/2, Sum25/2
  EnergyTotal/1 -> Sum20/2
  PI3/1 -> Gain1/1
  PI4/1 -> Gain43/1
  PI2/1 -> DiffabPowerRef/1
  PI10/1 -> DiffacPowerRef/1
  Gain43/1 -> Sum10/1
  Sum17/1 -> PI10/1
  Gain6/1 -> Sum17/1
  Sum10/1 -> PI2/1
  ACpowerFFd/1 -> Sum27/2
  Gain1/1 -> Sum27/1
  PI1/1 -> TotalPowerRef/1
  Sum27/1 -> PI1/1
  DiffacACpowerFFd/1 -> Sum17/2
  DiffabABpowerFFd/1 -> Sum10/2
  Mux/1 -> Scope/1

== system MTDC_MODEL/GRID3+MMC3/Feedforward calculation/First order filter1 ==
  In1 : Inport
  Demux11 : Demux  Outputs=3
  Mux23 : Mux  Inputs=3
  R1 : TransferFcn  Numerator=1  Denominator=[tau_isum 1]
  R2 : TransferFcn  Numerator=1  Denominator=[tau_isum 1]
  R3 : TransferFcn  Numerator=1  Denominator=[tau_isum 1]
  Out1 : Outport  VectorParamsAs1DForOutWhenUnconnected=off
  wires:
  Demux11/2 -> R2/1
  R2/1 -> Mux23/2  "Pub"
  Demux11/1 -> R1/1
  Demux11/3 -> R3/1
  Mux23/1 -> Out1/1
  In1/1 -> Demux11/1
  R3/1 -> Mux23/3  "Puc"
  R1/1 -> Mux23/1  "Pua"

== system MTDC_MODEL/GRID3+MMC3/Isum_AC_Ref_Cal/DIFFERENT_REF_CALC_METHODS  ==
  v_g_pos : Inport
  Constant{1..6} (6 alike) : Constant  Value=0
  Gain1 : Gain  Gain=1/sqrt(2)
  Gain13 : Gain  Gain=1/U_ll1
  Matrix Concatenate4 : Concatenate  NumInputs=3  Mode=Multidimensional array  ConcatenateDimension=2
  Memory : Memory  InitialCondition=Vpeak_d1
  Mux11 : Mux  Inputs=3
  Mux12 : Mux  Inputs=3
  Mux5 : Mux  Inputs=3
  inv mat2 : MATLAB Function  TreatAsAtomicUnit=on
  Initial Approach : Outport  VectorParamsAs1DForOutWhenUnconnected=off
  wires:
  Mux5/1 -> Matrix Concatenate4/3
  Mux11/1 -> Matrix Concatenate4/1
  Constant5/1 -> Mux11/2
  Matrix Concatenate4/1 -> inv mat2/1(u)  "Isum_neg; -Isum_neg;  Isum_pos"
  Constant4/1 -> Mux12/1
  [v_g_pos_rms_pu] -> Mux11/1
  [v_g_pos_rms_pu] -> Mux12/2
  Constant3/1 -> Mux5/2
  [v_g_pos_rms_pu] -> Mux5/3
  inv mat2/1(y) -> Initial Approach/1
  Mux12/1 -> Matrix Concatenate4/2
  Gain1/1 -> [v_g_pos_rms_pu]
  v_g_pos/1 -> Memory/1
  Gain13/1 -> Gain1/1
  Constant1/1 -> Mux11/3
  Constant2/1 -> Mux12/3
  Constant6/1 -> Mux5/1
  Memory/1 -> Gain13/1

== system MTDC_MODEL/GRID3+MMC3/Isum_AC_Ref_Cal/Rotation4 ==
  angle : Inport
  Gain1 : Gain
  Gain2 : Gain  Gain=-1
  Gain9 : Gain  Gain=-1
  Matrix Concatenate1 : Concatenate  Mode=Multidimensional array  ConcatenateDimension=2
  Matrix Concatenate2 : Concatenate  Mode=Multidimensional array  ConcatenateDimension=2
  Mux{1..2,8..9} (4 alike) : Mux  Inputs=2
  Trigonometric Function{1,3..4,6} (4 alike) : Trigonometry  Operator=cos
  Trigonometric Function{2,5,7..8} (4 alike) : Trigonometry
  iR : Outport  VectorParamsAs1DForOutWhenUnconnected=off
  R : Outport  Port=2  VectorParamsAs1DForOutWhenUnconnected=off
  wires:
  Gain2/1 -> Mux2/1
  Matrix Concatenate2/1 -> R/1
  Gain1/1 -> Mux1/2
  Mux2/1 -> Matrix Concatenate2/2
  Mux1/1 -> Matrix Concatenate2/1
  Trigonometric Function8/1 -> Gain2/1
  Trigonometric Function2/1 -> Gain1/1
  Trigonometric Function3/1 -> Mux2/2
  Trigonometric Function1/1 -> Mux1/1
  Matrix Concatenate1/1 -> iR/1
  Gain9/1 -> Mux8/2
  angle/1 -> Trigonometric Function1/1, Trigonometric Function2/1, Trigonometric Function8/1, Trigonometric Function3/1, Trigonometric Function4/1, Trigonometric Function5/1, Trigonometric Function7/1, Trigonometric Function6/1
  Mux9/1 -> Matrix Concatenate1/2
  Mux8/1 -> Matrix Concatenate1/1
  Trigonometric Function7/1 -> Mux9/1
  Trigonometric Function5/1 -> Gain9/1
  Trigonometric Function6/1 -> Mux9/2
  Trigonometric Function4/1 -> Mux8/1

== system MTDC_MODEL/GRID3+MMC3/vsum Calculation/PR Controller1 ==
  e : Inport
  PID Controller2 : pid_lib/PID Controller  Controller=PI  Form=Parallel  TimeDomain=Continuous-time  UseExternalTs=off  SampleTime=1  IntegratorMethod=Forward Euler  FilterMethod=Forward Euler  ControllerParametersSource=internal  P=Kp_sum  I=Ki_sum  D=0  UseFilter=on  N=100  TunerSelectOption=Transfer Function Based (PID Tuner App)  InitialConditionSource=internal  InitialConditionForIntegrator=0  InitialConditionForFilter=0  DifferentiatorICPrevScaledInput=0  ExternalReset=none  TrackingMode=off  Kt=1  LimitOutput=off  SatLimitsSource=internal  UpperSaturationLimit=inf  LowerSaturationLimit=-inf  LinearizeAsGain=on  AntiWindupMode=none  Kb=1  POutMin=[]  POutMax=[]  IOutMin=[]  IOutMax=[]  DOutMin=[]  DOutMax=[]  NOutMin=[]  NOutMax=[]  SumOutMin=[]  SumOutMax=[]  SaturationOutMin=[]  SaturationOutMax=[]  PParamMin=[]  PParamMax=[]  IParamMin=[]  IParamMax=[]  DParamMin=[]  DParamMax=[]  NParamMin=[]  NParamMax=[]  KbParamMin=[]  KbParamMax=[]  KtParamMin=[]  KtParamMax=[]  KbOutMin=[]  KbOutMax=[]  KtOutMin=[]  KtOutMax=[]  IntegratorOutMin=[]  IntegratorOutMax=[]  FilterOutMin=[]  FilterOutMax=[]  SumI1OutMin=[]  SumI1OutMax=[]  SumI2OutMin=[]  SumI2OutMax=[]  SumI3OutMin=[]  SumI3OutMax=[]  SumI4OutMin=[]  SumI4OutMax=[]  SumDOutMin=[]  SumDOutMax=[]  DifferentiatorOutMin=[]  DifferentiatorOutMax=[]  FilterDiffOutCoefMin=[]  FilterDiffOutCoefMax=[]  ReciprocalOutMin=[]  ReciprocalOutMax=[]  SumDenOutMin=[]  SumDenOutMax=[]  SumNumOutMin=[]  SumNumOutMax=[]  DivideOutMin=[]  DivideOutMax=[]  UdiffTsProdOutMin=[]  UdiffTsProdOutMax=[]  NTsProdOutMin=[]  NTsProdOutMax=[]  UintegralTsProdOutMin=[]  UintegralTsProdOutMax=[]  UngainTsProdOutMin=[]  UngainTsProdOutMax=[]  IntegratorContinuousStateAttributes=''  IntegratorStateMustResolveToSignalObject=off  IntegratorRTWStateStorageClass=Auto  FilterContinuousStateAttributes=''  FilterStateMustResolveToSignalObject=off  FilterRTWStateStorageClass=Auto  ParallelPVariant=InternalParameters  IdealPVariant=Disabled  IVariant=InternalParameters  DVariant=Disabled  IntegratorVariant=Continuous  SatVariant=Disabled  AWVariant=Passthrough  PCopyVariant=Disabled  TRVariant=Disabled  FdbkBlocksVariant=Forward  IdealPFdbkVariant=Disabled  SatFdbkVariant=Disabled  DerivativeFilterVariant=Disabled  NVariant=Disabled  NCopyVariant=Disabled_SignalSpec  FilterICVariant=Disabled  IntegratorICVariant=InternalICs  ExternalResetVariant=Disabled  TRSumVariant=Passthrough  SumFdbkVariant=Disabled  SumVariant=Sum_PI  TsampFilterVariant=InternalTs  TsampNgainVariant=Passthrough  TsampIntegralVariant=Passthrough  ExternalSaturationOutDataTypeStr=Inherit: Same as second input
  Sum1 : Sum  Inputs=++|
  Transfer Fcn : TransferFcn  Numerator=PR.num{1}  Denominator=PR.den{1}
  v : Outport
  wires:
  e/1 -> Transfer Fcn/1, PID Controller2/1
  Transfer Fcn/1 -> Sum1/2
  Sum1/1 -> v/1
  PID Controller2/1 -> Sum1/1

== system MTDC_MODEL/GRID3+MMC3/vsum Calculation/PR Controller2 ==
  e : Inport
  PID Controller2 : pid_lib/PID Controller  Controller=PI  Form=Parallel  TimeDomain=Continuous-time  UseExternalTs=off  SampleTime=1  IntegratorMethod=Forward Euler  FilterMethod=Forward Euler  ControllerParametersSource=internal  P=Kp_sum  I=Ki_sum  D=0  UseFilter=on  N=100  TunerSelectOption=Transfer Function Based (PID Tuner App)  InitialConditionSource=internal  InitialConditionForIntegrator=0  InitialConditionForFilter=0  DifferentiatorICPrevScaledInput=0  ExternalReset=none  TrackingMode=off  Kt=1  LimitOutput=off  SatLimitsSource=internal  UpperSaturationLimit=inf  LowerSaturationLimit=-inf  LinearizeAsGain=on  AntiWindupMode=none  Kb=1  POutMin=[]  POutMax=[]  IOutMin=[]  IOutMax=[]  DOutMin=[]  DOutMax=[]  NOutMin=[]  NOutMax=[]  SumOutMin=[]  SumOutMax=[]  SaturationOutMin=[]  SaturationOutMax=[]  PParamMin=[]  PParamMax=[]  IParamMin=[]  IParamMax=[]  DParamMin=[]  DParamMax=[]  NParamMin=[]  NParamMax=[]  KbParamMin=[]  KbParamMax=[]  KtParamMin=[]  KtParamMax=[]  KbOutMin=[]  KbOutMax=[]  KtOutMin=[]  KtOutMax=[]  IntegratorOutMin=[]  IntegratorOutMax=[]  FilterOutMin=[]  FilterOutMax=[]  SumI1OutMin=[]  SumI1OutMax=[]  SumI2OutMin=[]  SumI2OutMax=[]  SumI3OutMin=[]  SumI3OutMax=[]  SumI4OutMin=[]  SumI4OutMax=[]  SumDOutMin=[]  SumDOutMax=[]  DifferentiatorOutMin=[]  DifferentiatorOutMax=[]  FilterDiffOutCoefMin=[]  FilterDiffOutCoefMax=[]  ReciprocalOutMin=[]  ReciprocalOutMax=[]  SumDenOutMin=[]  SumDenOutMax=[]  SumNumOutMin=[]  SumNumOutMax=[]  DivideOutMin=[]  DivideOutMax=[]  UdiffTsProdOutMin=[]  UdiffTsProdOutMax=[]  NTsProdOutMin=[]  NTsProdOutMax=[]  UintegralTsProdOutMin=[]  UintegralTsProdOutMax=[]  UngainTsProdOutMin=[]  UngainTsProdOutMax=[]  IntegratorContinuousStateAttributes=''  IntegratorStateMustResolveToSignalObject=off  IntegratorRTWStateStorageClass=Auto  FilterContinuousStateAttributes=''  FilterStateMustResolveToSignalObject=off  FilterRTWStateStorageClass=Auto  ParallelPVariant=InternalParameters  IdealPVariant=Disabled  IVariant=InternalParameters  DVariant=Disabled  IntegratorVariant=Continuous  SatVariant=Disabled  AWVariant=Passthrough  PCopyVariant=Disabled  TRVariant=Disabled  FdbkBlocksVariant=Forward  IdealPFdbkVariant=Disabled  SatFdbkVariant=Disabled  DerivativeFilterVariant=Disabled  NVariant=Disabled  NCopyVariant=Disabled_SignalSpec  FilterICVariant=Disabled  IntegratorICVariant=InternalICs  ExternalResetVariant=Disabled  TRSumVariant=Passthrough  SumFdbkVariant=Disabled  SumVariant=Sum_PI  TsampFilterVariant=InternalTs  TsampNgainVariant=Passthrough  TsampIntegralVariant=Passthrough  ExternalSaturationOutDataTypeStr=Inherit: Same as second input
  Sum1 : Sum  Inputs=++|
  Transfer Fcn : TransferFcn  Numerator=PR.num{1}  Denominator=PR.den{1}
  v : Outport
  wires:
  PID Controller2/1 -> Sum1/1
  Sum1/1 -> v/1
  Transfer Fcn/1 -> Sum1/2
  e/1 -> PID Controller2/1, Transfer Fcn/1

== system MTDC_MODEL/GRID3+MMC3/vsum Calculation/PR Controller3 ==
  e : Inport
  PID Controller2 : pid_lib/PID Controller  Controller=PI  Form=Parallel  TimeDomain=Continuous-time  UseExternalTs=off  SampleTime=1  IntegratorMethod=Forward Euler  FilterMethod=Forward Euler  ControllerParametersSource=internal  P=Kp_sum  I=Ki_sum  D=0  UseFilter=on  N=100  TunerSelectOption=Transfer Function Based (PID Tuner App)  InitialConditionSource=internal  InitialConditionForIntegrator=0  InitialConditionForFilter=0  DifferentiatorICPrevScaledInput=0  ExternalReset=none  TrackingMode=off  Kt=1  LimitOutput=off  SatLimitsSource=internal  UpperSaturationLimit=inf  LowerSaturationLimit=-inf  LinearizeAsGain=on  AntiWindupMode=none  Kb=1  POutMin=[]  POutMax=[]  IOutMin=[]  IOutMax=[]  DOutMin=[]  DOutMax=[]  NOutMin=[]  NOutMax=[]  SumOutMin=[]  SumOutMax=[]  SaturationOutMin=[]  SaturationOutMax=[]  PParamMin=[]  PParamMax=[]  IParamMin=[]  IParamMax=[]  DParamMin=[]  DParamMax=[]  NParamMin=[]  NParamMax=[]  KbParamMin=[]  KbParamMax=[]  KtParamMin=[]  KtParamMax=[]  KbOutMin=[]  KbOutMax=[]  KtOutMin=[]  KtOutMax=[]  IntegratorOutMin=[]  IntegratorOutMax=[]  FilterOutMin=[]  FilterOutMax=[]  SumI1OutMin=[]  SumI1OutMax=[]  SumI2OutMin=[]  SumI2OutMax=[]  SumI3OutMin=[]  SumI3OutMax=[]  SumI4OutMin=[]  SumI4OutMax=[]  SumDOutMin=[]  SumDOutMax=[]  DifferentiatorOutMin=[]  DifferentiatorOutMax=[]  FilterDiffOutCoefMin=[]  FilterDiffOutCoefMax=[]  ReciprocalOutMin=[]  ReciprocalOutMax=[]  SumDenOutMin=[]  SumDenOutMax=[]  SumNumOutMin=[]  SumNumOutMax=[]  DivideOutMin=[]  DivideOutMax=[]  UdiffTsProdOutMin=[]  UdiffTsProdOutMax=[]  NTsProdOutMin=[]  NTsProdOutMax=[]  UintegralTsProdOutMin=[]  UintegralTsProdOutMax=[]  UngainTsProdOutMin=[]  UngainTsProdOutMax=[]  IntegratorContinuousStateAttributes=''  IntegratorStateMustResolveToSignalObject=off  IntegratorRTWStateStorageClass=Auto  FilterContinuousStateAttributes=''  FilterStateMustResolveToSignalObject=off  FilterRTWStateStorageClass=Auto  ParallelPVariant=InternalParameters  IdealPVariant=Disabled  IVariant=InternalParameters  DVariant=Disabled  IntegratorVariant=Continuous  SatVariant=Disabled  AWVariant=Passthrough  PCopyVariant=Disabled  TRVariant=Disabled  FdbkBlocksVariant=Forward  IdealPFdbkVariant=Disabled  SatFdbkVariant=Disabled  DerivativeFilterVariant=Disabled  NVariant=Disabled  NCopyVariant=Disabled_SignalSpec  FilterICVariant=Disabled  IntegratorICVariant=InternalICs  ExternalResetVariant=Disabled  TRSumVariant=Passthrough  SumFdbkVariant=Disabled  SumVariant=Sum_PI  TsampFilterVariant=InternalTs  TsampNgainVariant=Passthrough  TsampIntegralVariant=Passthrough  ExternalSaturationOutDataTypeStr=Inherit: Same as second input
  Sum1 : Sum  Inputs=++|
  Transfer Fcn : TransferFcn  Numerator=PR.num{1}  Denominator=PR.den{1}
  v : Outport
  wires:
  e/1 -> Transfer Fcn/1, PID Controller2/1
  Transfer Fcn/1 -> Sum1/2
  Sum1/1 -> v/1
  PID Controller2/1 -> Sum1/1

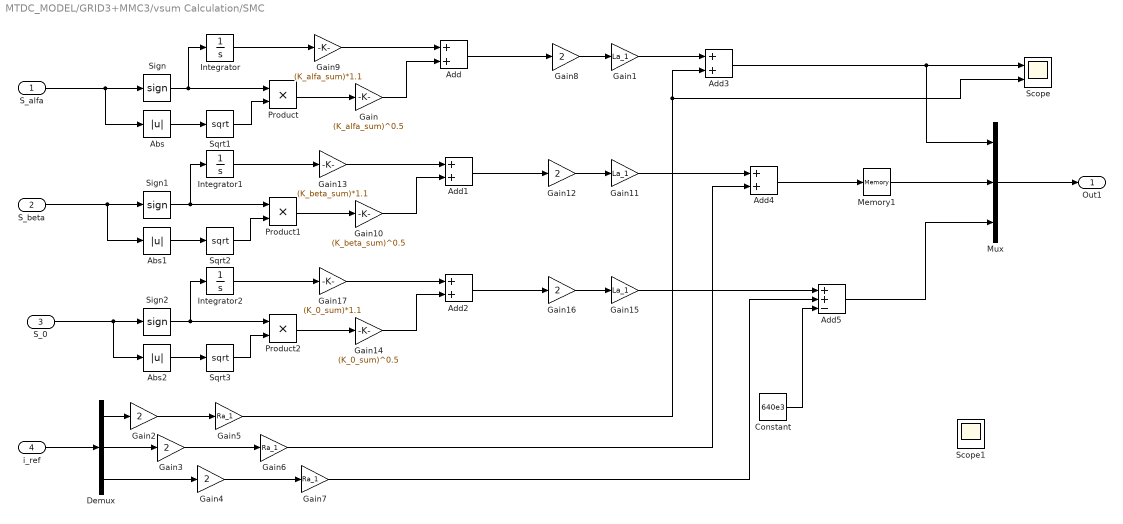
== system MTDC_MODEL/GRID3+MMC3/vsum Calculation/SMC ==
  S_alfa : Inport
  S_beta : Inport  Port=2
  S_0 : Inport  Port=3
  i_ref : Inport  Port=4
  Abs : Abs
  Abs1 : Abs
  Abs2 : Abs
  Add{,1..4} (5 alike) : Sum
  Add5 : Sum  Inputs=++-
  Constant : Constant  Value=640e3
  Demux : Demux  Outputs=3
  Gain : Gain  Gain=(K_alfa_sum)^0.5
  Gain1 : Gain  Gain=La_1
  Gain10 : Gain  Gain=(K_beta_sum)^0.5
  Gain11 : Gain  Gain=La_1
  Gain{2..4,8,12,16} (6 alike) : Gain  Gain=2
  Gain13 : Gain  Gain=(K_beta_sum)*1.1
  Gain14 : Gain  Gain=(K_0_sum)^0.5
  Gain15 : Gain  Gain=La_1
  Gain17 : Gain  Gain=(K_0_sum)*1.1
  Gain5 : Gain  Gain=Ra_1
  Gain6 : Gain  Gain=Ra_1
  Gain7 : Gain  Gain=Ra_1
  Gain9 : Gain  Gain=(K_alfa_sum)*1.1
  Integrator : Integrator
  Integrator1 : Integrator
  Integrator2 : Integrator
  Memory1 : Memory
  Mux : Mux  Inputs=3
  Product : Product
  Product1 : Product
  Product2 : Product
  Scope : Scope  NumInputPorts=2
  Scope1 : Scope
  Sign : Signum
  Sign1 : Signum
  Sign2 : Signum
  Sqrt1 : Sqrt  SaturateOnIntegerOverflow=on
  Sqrt2 : Sqrt  SaturateOnIntegerOverflow=on
  Sqrt3 : Sqrt  SaturateOnIntegerOverflow=on
  Out1 : Outport
  wires:
  i_ref/1 -> Demux/1
  Demux/1 -> Gain2/1
  Demux/2 -> Gain3/1
  Demux/3 -> Gain4/1
  Gain2/1 -> Gain5/1
  Gain3/1 -> Gain6/1
  Gain4/1 -> Gain7/1
  Gain8/1 -> Gain1/1
  S_alfa/1 -> Abs/1, Sign/1
  Sign/1 -> Integrator/1, Product/1
  Product/1 -> Gain/1
  Abs/1 -> Sqrt1/1
  Sqrt1/1 -> Product/2
  Integrator/1 -> Gain9/1
  Gain/1 -> Add/2
  Gain9/1 -> Add/1
  Add/1 -> Gain8/1
  Add1/1 -> Gain12/1
  Gain13/1 -> Add1/1
  Gain10/1 -> Add1/2
  Integrator1/1 -> Gain13/1
  Sqrt2/1 -> Product1/2
  Abs1/1 -> Sqrt2/1
  Product1/1 -> Gain10/1
  Sign1/1 -> Integrator1/1, Product1/1
  S_beta/1 -> Sign1/1, Abs1/1
  Gain12/1 -> Gain11/1
  Gain16/1 -> Gain15/1
  Sign2/1 -> Integrator2/1, Product2/1
  Product2/1 -> Gain14/1
  Abs2/1 -> Sqrt3/1
  Sqrt3/1 -> Product2/2
  Integrator2/1 -> Gain17/1
  Gain14/1 -> Add2/2
  Gain17/1 -> Add2/1
  Add2/1 -> Gain16/1
  Gain6/1 -> Add4/2
  Gain1/1 -> Add3/1
  Gain11/1 -> Add4/1
  Mux/1 -> Out1/1
  Add4/1 -> Memory1/1
  Add5/1 -> Mux/3
  Memory1/1 -> Mux/2
  Gain15/1 -> Add5/1
  Gain7/1 -> Add5/2
  Gain5/1 -> Scope/2, Add3/2
  Add3/1 -> Scope/1, Mux/1
  S_0/1 -> Abs2/1, Sign2/1
  Constant/1 -> Add5/3

== system MTDC_MODEL/GRID4+MMC4/Current loop1/PLCS ==
  iq : Inport
  Ref_iq : Inport  Port=2
  Ref_id : Inport  Port=3
  id : Inport  Port=4
  Abs2 : Abs
  Add : Sum  Inputs=---
  Add1 : Sum
  Constant : Constant  Value=-1/5
  Derivative : Derivative
  Gain1 : Gain  Gain=20000
  Gain14 : Gain  Gain=3900
  Gain2 : Gain  Gain=(Rg_1+Ra_1/2)
  Gain3 : Gain  Gain=(Lg_1+La_1/2)
  Gain6 : Gain  Gain=(Lg_1+La_1/2)*2*pi*50
  Power : Math  Operator=pow  SaturateOnIntegerOverflow=on
  Power1 : Math  Operator=pow  SaturateOnIntegerOverflow=on
  Product : Product
  Scope : Scope  NumInputPorts=2
  Sign1 : Signum
  Sign2 : Signum
  Sqrt3 : Sqrt  SaturateOnIntegerOverflow=on
  Sum5 : Sum  Inputs=|+-
  Out1 : Outport
  Sq : Outport  Port=2
  wires:
  Ref_id/1 -> Gain6/1
  Sum5/1 -> Sign1/1, Scope/2, Sq/1, Derivative/1, Abs2/1  "Sq"
  iq/1 -> Sum5/2
  Add/1 -> Out1/1
  Gain6/1 -> Add/1
  Gain2/1 -> Add/2
  Ref_iq/1 -> Gain2/1, Sum5/1
  Gain3/1 -> Scope/1, Add/3
  Abs2/1 -> Sqrt3/1
  Sign1/1 -> Product/1
  Sqrt3/1 -> Product/2
  Product/1 -> Gain14/1
  Gain14/1 -> Add1/1
  Derivative/1 -> Add1/2
  Add1/1 -> Sign2/1
  Gain1/1 -> Gain3/1
  Sign2/1 -> Gain1/1

== system MTDC_MODEL/GRID4+MMC4/Current loop1/SMC ==
  iq : Inport
  Ref_iq : Inport  Port=2
  Ref_id : Inport  Port=3
  id : Inport  Port=4
  Add : Sum  Inputs=---
  Gain2 : Gain  Gain=(Rg_1+Ra_1/2)
  Gain3 : Gain  Gain=Kq
  Gain4 : Gain  Gain=Qq
  Gain5 : Gain  Gain=(Lg_1+La_1/2)
  Gain6 : Gain  Gain=(Lg_1+La_1/2)*2*pi*50
  Sign : Signum  ZeroCross=off
  Sum2 : Sum  Inputs=|++
  Sum5 : Sum  Inputs=|+-
  Out1 : Outport
  wires:
  Ref_id/1 -> Gain6/1
  Sum5/1 -> Sign/1, Gain3/1  "Sq"
  iq/1 -> Sum5/2
  Add/1 -> Out1/1
  Gain6/1 -> Add/1
  Gain2/1 -> Add/2
  Gain5/1 -> Add/3
  Ref_iq/1 -> Sum5/1, Gain2/1
  Sum2/1 -> Gain5/1
  Gain4/1 -> Sum2/1
  Gain3/1 -> Sum2/2
  Sign/1 -> Gain4/1
